simulink model "Flight_Simulation"  (R2021b)
settings: Solver=ode4  StartTime=0.0  StopTime=20  FixedStep=Settings.Simulation.step_size  RelTol=1e-3  EnableMultiTasking=on
undefined symbols (not defined in the file or in its folder): AeroCoeff, Aircraft, ControlGains, dLEF, Environment, F, Light, MIL, Settings, Trim, trim_control, trim_state, trim_thrust
libraries: simulink x19, simulink_extras x14, slpidlib x2, aerolibfltsims x2, aerolibwind2 x1, vrlib x1
(part 2 of 5)

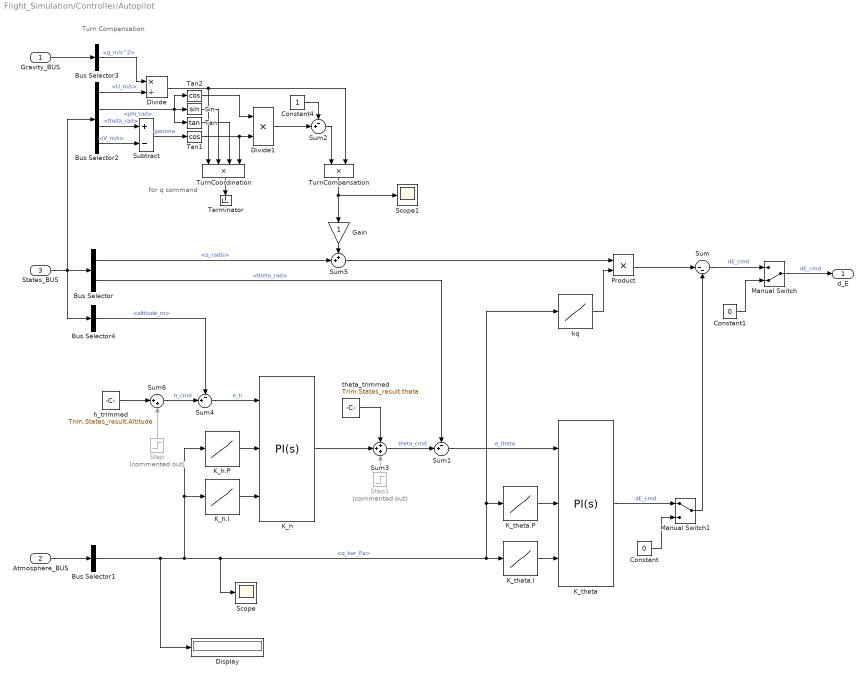
== system Flight_Simulation/Controller/Autopilot ==
  note: for q command
  note: Turn Compensation
  Gravity_BUS : Inport
  Atmosphere_BUS : Inport  Port=2
  States_BUS : Inport  Port=3
  Bus Selector : BusSelector  OutputSignals=Rates_p_q_r.q_rad/s,Angles_phi_theta_psi.theta_rad
  Bus Selector1 : BusSelector  OutputSignals=q_bar_Pa
  Bus Selector2 : BusSelector  OutputSignals=Vel_U_V_W_body.U_m/s,Angles_phi_theta_psi.phi_rad,Angles_phi_theta_psi.theta_rad,Vel_U_V_W_body.V_m/s
  Bus Selector3 : BusSelector  OutputSignals=g_m/s^2
  Bus Selector4 : BusSelector  OutputSignals=Position_north_east_alt.altitude_m
  Constant : Constant  Value=0
  Constant1 : Constant  Value=0
  Constant4 : Constant
  Display : Display
  Divide : Product  Inputs=*/
  Divide1 : Product  Inputs=**
  Gain : Gain
  K_h : slpidlib/PID Controller  Controller=PI  Form=Parallel  TimeDomain=Continuous-time  UseExternalTs=off  SampleTime=-1  IntegratorMethod=Forward Euler  FilterMethod=Forward Euler  ControllerParametersSource=external  P=1  I=1  D=0  UseFilter=on  N=100  TunerSelectOption=Transfer Function Based (PID Tuner App)  InitialConditionSource=internal  InitialConditionForIntegrator=0  InitialConditionForFilter=0  DifferentiatorICPrevScaledInput=0  ExternalReset=none  TrackingMode=off  Kt=1  LimitOutput=off  SatLimitsSource=internal  UpperSaturationLimit=inf  LowerSaturationLimit=-inf  LinearizeAsGain=on  AntiWindupMode=none  Kb=1  POutMin=[]  POutMax=[]  IOutMin=[]  IOutMax=[]  DOutMin=[]  DOutMax=[]  NOutMin=[]  NOutMax=[]  SumOutMin=[]  SumOutMax=[]  SaturationOutMin=[]  SaturationOutMax=[]  PParamMin=[]  PParamMax=[]  IParamMin=[]  IParamMax=[]  DParamMin=[]  DParamMax=[]  NParamMin=[]  NParamMax=[]  KbParamMin=[]  KbParamMax=[]  KtParamMin=[]  KtParamMax=[]  KbOutMin=[]  KbOutMax=[]  KtOutMin=[]  KtOutMax=[]  IntegratorOutMin=[]  IntegratorOutMax=[]  FilterOutMin=[]  FilterOutMax=[]  SumI1OutMin=[]  SumI1OutMax=[]  SumI2OutMin=[]  SumI2OutMax=[]  SumI3OutMin=[]  SumI3OutMax=[]  SumI4OutMin=[]  SumI4OutMax=[]  SumDOutMin=[]  SumDOutMax=[]  DifferentiatorOutMin=[]  DifferentiatorOutMax=[]  FilterDiffOutCoefMin=[]  FilterDiffOutCoefMax=[]  ReciprocalOutMin=[]  ReciprocalOutMax=[]  SumDenOutMin=[]  SumDenOutMax=[]  SumNumOutMin=[]  SumNumOutMax=[]  DivideOutMin=[]  DivideOutMax=[]  UdiffTsProdOutMin=[]  UdiffTsProdOutMax=[]  NTsProdOutMin=[]  NTsProdOutMax=[]  UintegralTsProdOutMin=[]  UintegralTsProdOutMax=[]  UngainTsProdOutMin=[]  UngainTsProdOutMax=[]  IntegratorContinuousStateAttributes=''  IntegratorStateMustResolveToSignalObject=off  IntegratorRTWStateStorageClass=Auto  FilterContinuousStateAttributes=''  FilterStateMustResolveToSignalObject=off  FilterRTWStateStorageClass=Auto  ParallelPVariant=ExternalParameters  IdealPVariant=Disabled  IVariant=ExternalParameters  DVariant=Disabled  IntegratorVariant=Continuous  SatVariant=Disabled  AWVariant=Passthrough  PCopyVariant=Disabled  TRVariant=Disabled  FdbkBlocksVariant=Forward  IdealPFdbkVariant=Disabled  SatFdbkVariant=Disabled  DerivativeFilterVariant=Disabled  NVariant=Disabled  NCopyVariant=Disabled_SignalSpec  FilterICVariant=Disabled  IntegratorICVariant=InternalICs  ExternalResetVariant=Disabled  TRSumVariant=Passthrough  SumFdbkVariant=Disabled  SumVariant=Sum_PI  TsampFilterVariant=InternalTs  TsampNgainVariant=Passthrough  TsampIntegralVariant=Passthrough  ExternalSaturationOutDataTypeStr=Inherit: Same as second input
  K_h.I : Lookup_n-D  NumberOfTableDimensions=1  BreakpointsForDimension1=ControlGains.Schedule  Table=ControlGains.K_h.I  InternalRulePriority=Speed  RndMeth=Simplest  InputSameDT=on
  K_h.P : Lookup_n-D  NumberOfTableDimensions=1  BreakpointsForDimension1=ControlGains.Schedule  Table=ControlGains.K_h.P  InternalRulePriority=Speed  RndMeth=Simplest  InputSameDT=on
  K_theta : slpidlib/PID Controller  Controller=PI  Form=Parallel  TimeDomain=Continuous-time  UseExternalTs=off  SampleTime=-1  IntegratorMethod=Forward Euler  FilterMethod=Forward Euler  ControllerParametersSource=external  P=1  I=1  D=0  UseFilter=on  N=100  TunerSelectOption=Transfer Function Based (PID Tuner App)  InitialConditionSource=internal  InitialConditionForIntegrator=0  InitialConditionForFilter=0  DifferentiatorICPrevScaledInput=0  ExternalReset=none  TrackingMode=off  Kt=1  LimitOutput=off  SatLimitsSource=internal  UpperSaturationLimit=inf  LowerSaturationLimit=-inf  LinearizeAsGain=on  AntiWindupMode=none  Kb=1  POutMin=[]  POutMax=[]  IOutMin=[]  IOutMax=[]  DOutMin=[]  DOutMax=[]  NOutMin=[]  NOutMax=[]  SumOutMin=[]  SumOutMax=[]  SaturationOutMin=[]  SaturationOutMax=[]  PParamMin=[]  PParamMax=[]  IParamMin=[]  IParamMax=[]  DParamMin=[]  DParamMax=[]  NParamMin=[]  NParamMax=[]  KbParamMin=[]  KbParamMax=[]  KtParamMin=[]  KtParamMax=[]  KbOutMin=[]  KbOutMax=[]  KtOutMin=[]  KtOutMax=[]  IntegratorOutMin=[]  IntegratorOutMax=[]  FilterOutMin=[]  FilterOutMax=[]  SumI1OutMin=[]  SumI1OutMax=[]  SumI2OutMin=[]  SumI2OutMax=[]  SumI3OutMin=[]  SumI3OutMax=[]  SumI4OutMin=[]  SumI4OutMax=[]  SumDOutMin=[]  SumDOutMax=[]  DifferentiatorOutMin=[]  DifferentiatorOutMax=[]  FilterDiffOutCoefMin=[]  FilterDiffOutCoefMax=[]  ReciprocalOutMin=[]  ReciprocalOutMax=[]  SumDenOutMin=[]  SumDenOutMax=[]  SumNumOutMin=[]  SumNumOutMax=[]  DivideOutMin=[]  DivideOutMax=[]  UdiffTsProdOutMin=[]  UdiffTsProdOutMax=[]  NTsProdOutMin=[]  NTsProdOutMax=[]  UintegralTsProdOutMin=[]  UintegralTsProdOutMax=[]  UngainTsProdOutMin=[]  UngainTsProdOutMax=[]  IntegratorContinuousStateAttributes=''  IntegratorStateMustResolveToSignalObject=off  IntegratorRTWStateStorageClass=Auto  FilterContinuousStateAttributes=''  FilterStateMustResolveToSignalObject=off  FilterRTWStateStorageClass=Auto  ParallelPVariant=ExternalParameters  IdealPVariant=Disabled  IVariant=ExternalParameters  DVariant=Disabled  IntegratorVariant=Continuous  SatVariant=Disabled  AWVariant=Passthrough  PCopyVariant=Disabled  TRVariant=Disabled  FdbkBlocksVariant=Forward  IdealPFdbkVariant=Disabled  SatFdbkVariant=Disabled  DerivativeFilterVariant=Disabled  NVariant=Disabled  NCopyVariant=Disabled_SignalSpec  FilterICVariant=Disabled  IntegratorICVariant=InternalICs  ExternalResetVariant=Disabled  TRSumVariant=Passthrough  SumFdbkVariant=Disabled  SumVariant=Sum_PI  TsampFilterVariant=InternalTs  TsampNgainVariant=Passthrough  TsampIntegralVariant=Passthrough  ExternalSaturationOutDataTypeStr=Inherit: Same as second input
  K_theta.I : Lookup_n-D  NumberOfTableDimensions=1  BreakpointsForDimension1=ControlGains.Schedule  Table=ControlGains.K_theta.I  InternalRulePriority=Speed  RndMeth=Simplest  InputSameDT=on
  K_theta.P : Lookup_n-D  NumberOfTableDimensions=1  BreakpointsForDimension1=ControlGains.Schedule  Table=ControlGains.K_theta.P  InternalRulePriority=Speed  RndMeth=Simplest  InputSameDT=on
  Manual Switch : ManualSwitch  CurrentSetting=0
  Manual Switch1 : ManualSwitch
  Product : Product
  Scope : Scope
  Scope1 : Scope
  Sin : Trigonometry
  Step : Step  Commented=on  Time=5  After=10  SampleTime=0
  Step1 : Step  Commented=on  Time=5  After=1*pi/180  SampleTime=0
  Subtract : Sum  Inputs=+-
  Sum : Sum  Inputs=|--
  Sum1 : Sum  Inputs=-+|
  Sum2 : Sum  Inputs=-+|
  Sum3 : Sum  Inputs=+++
  Sum4 : Sum  Inputs=-+|
  Sum5 : Sum  Inputs=++|
  Sum6 : Sum  Inputs=|++
  Tan : Trigonometry  Operator=tan
  Tan1 : Trigonometry  Operator=cos
  Tan2 : Trigonometry  Operator=cos
  Terminator : Terminator
  TurnCompensation : Product
  TurnCoordination : Product  Inputs=4
  h_trimmed : Constant  Value=Trim.States_result.Altitude
  kq : Lookup_n-D  NumberOfTableDimensions=1  BreakpointsForDimension1=ControlGains.Schedule  Table=ControlGains.kq  InternalRulePriority=Speed  RndMeth=Simplest  InputSameDT=on
  theta_trimmed : Constant  Value=Trim.States_result.theta
  d_E : Outport
  wires:
  States_BUS/1 -> Bus Selector2/1, Bus Selector4/1, Bus Selector/1
  Product/1 -> Sum/1
  Manual Switch/1 -> d_E/1  "dE_cmd"
  Sum/1 -> Manual Switch/1  "dE_cmd"
  Constant/1 -> Manual Switch1/2
  Manual Switch1/1 -> Sum/2
  Constant1/1 -> Manual Switch/2
  Sum1/1 -> K_theta/1  "e_theta"
  Bus Selector2/1 -> Divide/2  "<U_m/s>"
  Gravity_BUS/1 -> Bus Selector3/1
  Bus Selector3/1 -> Divide/1  "<g_m/s^2>"
  Divide/1 -> TurnCompensation/2, TurnCoordination/1
  Bus Selector2/2 -> Tan2/1, Sin/1, Tan/1  "<phi_rad>"
  Bus Selector2/4 -> Subtract/2  "<V_m/s>"
  Bus Selector2/3 -> Subtract/1  "<theta_rad>"
  TurnCoordination/1 -> Terminator/1
  Step1/1 -> Sum3/3
  Subtract/1 -> Tan1/1  "gamma"
  Tan1/1 -> Divide1/2, TurnCoordination/4
  Tan/1 -> TurnCoordination/3
  Sin/1 -> TurnCoordination/2
  Atmosphere_BUS/1 -> Bus Selector1/1
  theta_trimmed/1 -> Sum3/1
  Bus Selector4/1 -> Sum4/1  "<altitude_m>"
  h_trimmed/1 -> Sum6/1
  Sum4/1 -> K_h/1  "e_h"
  Step/1 -> Sum6/2
  Bus Selector/1 -> Sum5/2  "<q_rad/s>"
  Bus Selector/2 -> Sum1/1  "<theta_rad>"
  Constant4/1 -> Sum2/1
  Divide1/1 -> Sum2/2
  Sum2/1 -> TurnCompensation/1
  Sum5/1 -> Product/1
  Tan2/1 -> Divide1/1
  TurnCompensation/1 -> Gain/1, Scope1/1
  K_theta/1 -> Manual Switch1/1  "dE_cmd"
  K_h/1 -> Sum3/2
  Sum3/1 -> Sum1/2  "theta_cmd"
  Sum6/1 -> Sum4/2  "h_cmd"
  Bus Selector1/1 -> Display/1, K_h.I/1, K_h.P/1, Scope/1, kq/1, K_theta.P/1, K_theta.I/1  "<q_bar_Pa>"
  kq/1 -> Product/2
  K_h.P/1 -> K_h/2
  K_h.I/1 -> K_h/3
  K_theta.P/1 -> K_theta/2
  K_theta.I/1 -> K_theta/3
  Gain/1 -> Sum5/1

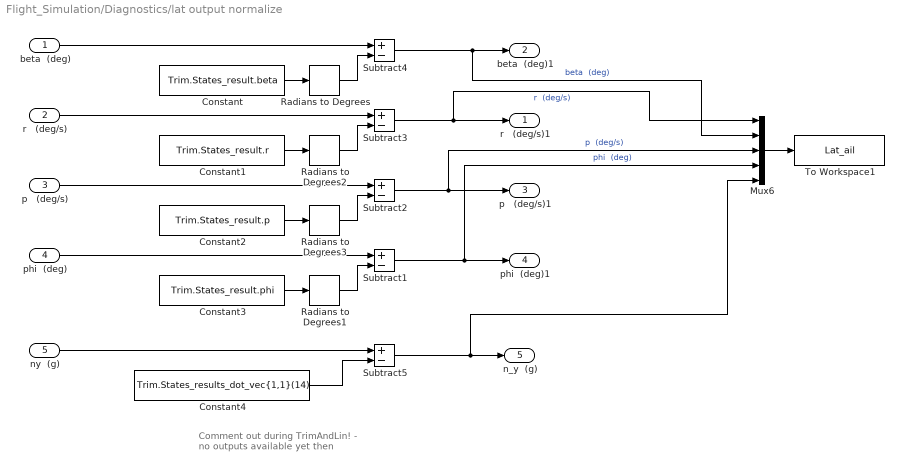
== system Flight_Simulation/Diagnostics/lat output normalize ==
  note: Comment out during TrimAndLin!
      | - no outputs available yet then
  beta  (deg) : Inport
  r   (deg/s) : Inport  Port=2
  p   (deg/s) : Inport  Port=3
  phi  (deg) : Inport  Port=4
  ny  (g) : Inport  Port=5
  Constant : Constant  Value=Trim.States_result.beta
  Constant1 : Constant  Value=Trim.States_result.r
  Constant2 : Constant  Value=Trim.States_result.p
  Constant3 : Constant  Value=Trim.States_result.phi
  Constant4 : Constant  Value=Trim.States_results_dot_vec{1,1}(14)
  Mux6 : Mux  Inputs=5
  Radians to Degrees{,1..3} (4 alike) : simulink_extras/Transformations/Radians to Degrees
  Subtract{1..5} (5 alike) : Sum  Inputs=+-
  To Workspace1 : ToWorkspace  VariableName=Lat_ail  SampleTime=-1
  r   (deg/s)1 : Outport
  beta  (deg)1 : Outport  Port=2
  p   (deg/s)1 : Outport  Port=3
  phi  (deg)1 : Outport  Port=4
  n_y  (g) : Outport  Port=5
  wires:
  beta  (deg)/1 -> Subtract4/1
  p   (deg/s)/1 -> Subtract2/1
  r   (deg/s)/1 -> Subtract3/1
  phi  (deg)/1 -> Subtract1/1
  Constant/1 -> Radians to Degrees/1
  Constant1/1 -> Radians to Degrees2/1
  Constant2/1 -> Radians to Degrees3/1
  Constant3/1 -> Radians to Degrees1/1
  Radians to Degrees/1 -> Subtract4/2
  Radians to Degrees2/1 -> Subtract3/2
  Radians to Degrees3/1 -> Subtract2/2
  Radians to Degrees1/1 -> Subtract1/2
  Constant4/1 -> Subtract5/2
  ny  (g)/1 -> Subtract5/1
  Subtract4/1 -> Mux6/2, beta  (deg)1/1  "beta  (deg)"
  Subtract3/1 -> Mux6/1, r   (deg/s)1/1  "r  (deg/s)"
  Subtract1/1 -> Mux6/4, phi  (deg)1/1  "phi  (deg)"
  Subtract2/1 -> Mux6/3, p   (deg/s)1/1  "p  (deg/s)"
  Mux6/1 -> To Workspace1/1
  Subtract5/1 -> Mux6/5, n_y  (g)/1

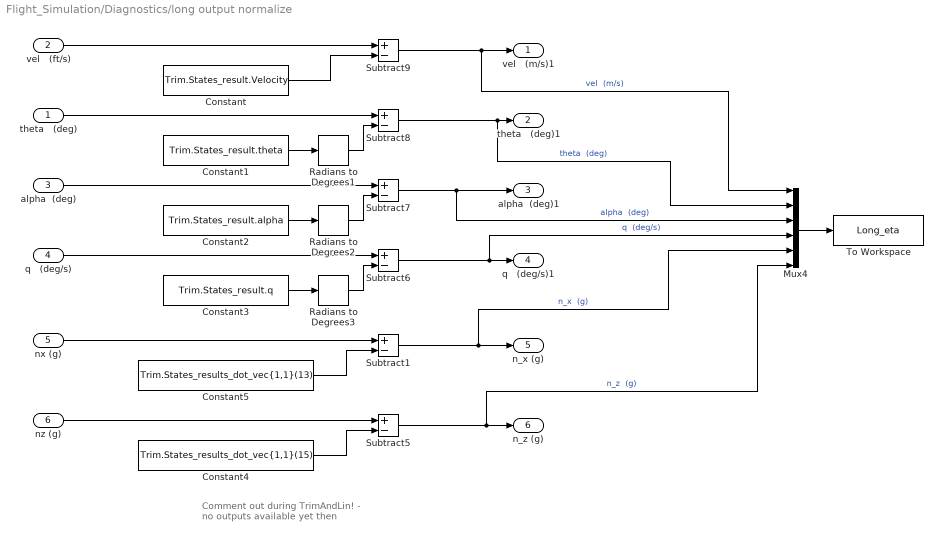
== system Flight_Simulation/Diagnostics/long output normalize ==
  note: Comment out during TrimAndLin!
      | - no outputs available yet then
  theta   (deg) : Inport
  vel   (ft/s) : Inport  Port=2
  alpha  (deg) : Inport  Port=3
  q   (deg/s) : Inport  Port=4
  nx (g) : Inport  Port=5
  nz (g) : Inport  Port=6
  Constant : Constant  Value=Trim.States_result.Velocity
  Constant1 : Constant  Value=Trim.States_result.theta
  Constant2 : Constant  Value=Trim.States_result.alpha
  Constant3 : Constant  Value=Trim.States_result.q
  Constant4 : Constant  Value=Trim.States_results_dot_vec{1,1}(15)
  Constant5 : Constant  Value=Trim.States_results_dot_vec{1,1}(13)
  Mux4 : Mux  Inputs=6
  Radians to Degrees1 : simulink_extras/Transformations/Radians to Degrees
  Radians to Degrees2 : simulink_extras/Transformations/Radians to Degrees
  Radians to Degrees3 : simulink_extras/Transformations/Radians to Degrees
  Subtract{1,5..9} (6 alike) : Sum  Inputs=+-
  To Workspace : ToWorkspace  VariableName=Long_eta  SampleTime=-1
  vel   (m/s)1 : Outport
  theta   (deg)1 : Outport  Port=2
  alpha  (deg)1 : Outport  Port=3
  q   (deg/s)1 : Outport  Port=4
  n_x (g) : Outport  Port=5
  n_z (g) : Outport  Port=6
  wires:
  vel   (ft/s)/1 -> Subtract9/1
  alpha  (deg)/1 -> Subtract7/1
  theta   (deg)/1 -> Subtract8/1
  nz (g)/1 -> Subtract5/1
  q   (deg/s)/1 -> Subtract6/1
  Constant/1 -> Subtract9/2
  Constant1/1 -> Radians to Degrees1/1
  Constant2/1 -> Radians to Degrees2/1
  Constant3/1 -> Radians to Degrees3/1
  Constant4/1 -> Subtract5/2
  Radians to Degrees1/1 -> Subtract8/2
  Radians to Degrees2/1 -> Subtract7/2
  Radians to Degrees3/1 -> Subtract6/2
  Constant5/1 -> Subtract1/2
  nx (g)/1 -> Subtract1/1
  Subtract7/1 -> Mux4/3, alpha  (deg)1/1  "alpha  (deg)"
  Subtract5/1 -> Mux4/6, n_z (g)/1  "n_z  (g)"
  Subtract8/1 -> Mux4/2, theta   (deg)1/1  "theta  (deg)"
  Mux4/1 -> To Workspace/1
  Subtract1/1 -> Mux4/5, n_x (g)/1  "n_x  (g)"
  Subtract6/1 -> Mux4/4, q   (deg/s)1/1  "q  (deg/s)"
  Subtract9/1 -> Mux4/1, vel   (m/s)1/1  "vel  (m/s)"

== system Flight_Simulation/Environment_Subsystems/Earth_Model ==
  States_BUS : Inport
  Bus Creator : BusCreator  Inputs=3
  Bus Selector : BusSelector  OutputSignals=Pos_WGS84.mue_pos_WGS84_rad
  Constant : Constant
  Earth_Radius_m : Constant  Value=6371000
  Earth_rotation_rate_rad/s : Constant  Commented=on  Value=7.2921150e-5
  Math Function : Math  Operator=square  SignedPower=on  SaturateOnIntegerOverflow=on
  Product : Product
  Product1 : Product  Inputs=*/
  Product2 : Product  Inputs=*/*
  Semi_major_axis_m : Constant  Value=6378137
  Sqrt : Sqrt  SaturateOnIntegerOverflow=on
  Sum : Sum  Inputs=|-+
  Sum1 : Sum  Inputs=+-|
  Terminator : Terminator
  Trigonometric Function : Trigonometry
  first_excentricity_squared : Constant  Value=6.69437999014*10^(-3)
  Earth_Model_BUS : Outport
  wires:
  Trigonometric Function/1 -> Math Function/1
  Math Function/1 -> Product/1
  first_excentricity_squared/1 -> Sum1/2, Product/2
  Product/1 -> Sum/1
  Constant/1 -> Sum1/1, Sum/2
  Sum/1 -> Product2/2, Sqrt/1
  Sqrt/1 -> Product1/2
  Semi_major_axis_m/1 -> Product1/1
  Sum1/1 -> Product2/3
  Product1/1 -> Product2/1, Bus Creator/1  "R_Curvature_Prime_Vertical_m"
  Earth_Radius_m/1 -> Terminator/1  "round_earth"
  Product2/1 -> Bus Creator/2  "R_Curvature_Meridian_m"
  Bus Creator/1 -> Earth_Model_BUS/1  "Earth_Model_BUS"
  Earth_rotation_rate_rad/s/1 -> Bus Creator/3  "Earth_rotation_rate_rad/s"
  States_BUS/1 -> Bus Selector/1  "Pos_mue_WGS84"
  Bus Selector/1 -> Trigonometric Function/1  "<mue_pos_WGS84_rad>"

== system Flight_Simulation/Environment_Subsystems/Gravity_Model_simple ==
  States_BUS : Inport
  Bus Creator : BusCreator  Inputs=1
  Terminator : Terminator
  g : Constant  Value=Environment.Const.g0
  Gravity_BUS : Outport
  wires:
  States_BUS/1 -> Terminator/1
  g/1 -> Bus Creator/1  "g_m/s^2"
  Bus Creator/1 -> Gravity_BUS/1  "Gravity_BUS"

== system Flight_Simulation/Environment_Subsystems/ISA_StandardAtmosphere_Model_ScriptVersion ==
  States_BUS : Inport
  Gravity_BUS : Inport  Port=2
  Vel_Aero_BUS : Inport  Port=3
  Bus Creator : BusCreator  Inputs=5
  Bus Selector : BusSelector  OutputSignals=Position_north_east_alt.altitude_m
  Bus Selector1 : BusSelector  OutputSignals=g_m/s^2
  Bus Selector2 : BusSelector  OutputSignals=Vel_aero_V_alpha_beta.v_m/s
  Compressibility_Setting : Constant  Value=Settings.Compressibility
  ISA_Standard_Atmosphere_Model : MATLAB Function  TreatAsAtomicUnit=on
  R : Constant  Value=Environment.Const.R
  Atmosphere_BUS : Outport
  wires:
  States_BUS/1 -> Bus Selector/1
  Bus Creator/1 -> Atmosphere_BUS/1  "Atmosphere_BUS"
  Bus Selector/1 -> ISA_Standard_Atmosphere_Model/1(H)  "<altitude_m>"
  Gravity_BUS/1 -> Bus Selector1/1
  Bus Selector1/1 -> ISA_Standard_Atmosphere_Model/3(g)  "<g_m/s^2>"
  ISA_Standard_Atmosphere_Model/3(rho) -> Bus Creator/3  "rho_kg/m^3"
  ISA_Standard_Atmosphere_Model/4(T) -> Bus Creator/4  "T_K"
  ISA_Standard_Atmosphere_Model/5(Mach) -> Bus Creator/5  "Mach"
  ISA_Standard_Atmosphere_Model/2(q_bar) -> Bus Creator/2  "q_bar_Pa"
  ISA_Standard_Atmosphere_Model/1(p_static) -> Bus Creator/1  "p_static_Pa"
  R/1 -> ISA_Standard_Atmosphere_Model/4(R)
  Compressibility_Setting/1 -> ISA_Standard_Atmosphere_Model/5(compressibility)
  Vel_Aero_BUS/1 -> Bus Selector2/1
  Bus Selector2/1 -> ISA_Standard_Atmosphere_Model/2(V)  "<v_m/s>"

== system Flight_Simulation/Environment_Subsystems/ISA_StandardAtmosphere_Model_SimulinkVersion ==
  note: to be updated
  States_BUS : Inport
  Gravity_BUS : Inport  Port=2
  Vel_aero_BUS : Inport  Port=3
  Bus Creator : BusCreator  Inputs=5
  Bus Selector : BusSelector  OutputSignals=Position_north_east_alt.altitude_m
  Bus Selector1 : BusSelector  OutputSignals=g_m/s^2
  Bus Selector2 : BusSelector  OutputSignals=Vel_aero_V_alpha_beta.v_m/s
  Constants depending on Height : Subsystem
  Divide1 : Product  Inputs=/*
  Gain : Gain  Gain=-1
  Height flags : Subsystem
  Mach : Subsystem
  T : Subsystem
  p_static : Subsystem
  q_bar : Subsystem
  rho : Subsystem
  Atmosphere_BUS : Outport
  wires:
  States_BUS/1 -> Bus Selector/1
  Bus Selector/1 -> Height flags/1(altitude), Constants depending on Height/1(altitude)  "<altitude_m>"
  Bus Creator/1 -> Atmosphere_BUS/1  "Atmosphere_BUS"
  Bus Selector2/1 -> q_bar/3(v), Mach/3(v)  "<v_m/s>"
  p_static/1(p) -> q_bar/1(p_static), Bus Creator/1  "p_static_Pa"
  Height flags/1(Height_flg) -> T/3(Height_flg), p_static/6(Height_flg), rho/6(Height_flg), Constants depending on Height/2(Height_flg)
  Constants depending on Height/5((H - H_A)*beta) -> T/1((H - H_A)*beta), rho/4((H - H_A)*beta), p_static/4((H - H_A)*beta)
  Mach/1(Mach) -> q_bar/4(Mach), Bus Creator/5  "Mach"
  q_bar/1(q_bar) -> Bus Creator/2  "q_bar_Pa"
  T/1(T) -> Bus Creator/4, Mach/1(T)  "T_K"
  rho/1(rho) -> Bus Creator/3, q_bar/2(rho)  "rho_kg/m^3"
  Constants depending on Height/4(H - H_A) -> p_static/3(H - H_A), rho/3(H - H_A)
  Gravity_BUS/1 -> Bus Selector1/1
  Bus Selector1/1 -> Divide1/2  "<g_m/s^2>"
  Divide1/1 -> Gain/1  "g/R"
  Gain/1 -> p_static/7(-g/R), rho/7(-g/R)  "-g/R"
  Constants depending on Height/6(T_A) -> p_static/5(T_A), T/2(T_A), rho/5(T_A)
  Constants depending on Height/1(p_A) -> p_static/1(p_A)
  Constants depending on Height/7(R) -> Mach/2(R), Divide1/1
  Constants depending on Height/2(rho_A) -> rho/1(rho_A)
  Constants depending on Height/3(beta) -> p_static/2(beta), rho/2(beta)
  Vel_aero_BUS/1 -> Bus Selector2/1

== system Flight_Simulation/Environment_Subsystems/Wind_Input ==
  States_BUS : Inport
  Wind_BUS : Inport  Port=2
  Flag_Settings_BUS : Inport  Port=3
  Const_Wind_Vel_UVWe_m/s : Inport  Port=4
  Bus Creator : BusCreator  Inputs=2
  Bus Creator1 : BusCreator  Inputs=3
  Bus Selector : BusSelector  OutputSignals=Angles_phi_theta_psi,Vel_U_V_W_body
  Bus Selector1 : BusSelector  OutputSignals=u_wind_m/s,v_wind_m/s,w_wind_m/s
  Bus Selector2 : BusSelector  OutputSignals=U_m/s,V_m/s,W_m/s
  Bus Selector3 : BusSelector  OutputSignals=phi_rad,theta_rad,psi_rad
  Bus Selector4 : BusSelector  OutputSignals=const_u_wind_m/s,const_v_wind_m/s,const_w_wind_m/s
  Bypass for TrimAndLin : Subsystem
  Calc_Vel_aero_alpha_beta : Subsystem
  Sum : Sum  Inputs=-+|
  Sum1 : Sum  Inputs=-+|
  Sum2 : Sum  Inputs=++|
  Sum3 : Sum  Inputs=++|
  Sum4 : Sum  Inputs=++|
  Sum5 : Sum  Inputs=-+|
  wind earth2body trafo : MATLAB Function  TreatAsAtomicUnit=on
  Vel_aero_BUS : Outport
  wires:
  States_BUS/1 -> Bus Selector/1
  Bus Selector/1 -> Bus Selector3/1  "<Angles_phi_theta_psi>"
  Bus Creator/1 -> Vel_aero_BUS/1  "Vel_aero_BUS"
  Wind_BUS/1 -> Bypass for TrimAndLin/1(Wind_BUS)
  Bus Selector1/1 -> Sum3/2  "<u_wind_m/s>"
  Bus Selector1/2 -> Sum4/2  "<v_wind_m/s>"
  Bus Selector1/3 -> Sum2/2  "<w_wind_m/s>"
  Bus Selector3/1 -> wind earth2body trafo/4(phi)  "<phi_rad>"
  Bus Selector3/2 -> wind earth2body trafo/5(theta)  "<theta_rad>"
  Bus Selector3/3 -> wind earth2body trafo/6(psi)  "<psi_rad>"
  Const_Wind_Vel_UVWe_m/s/1 -> Bus Selector4/1
  Bus Selector4/3 -> Sum2/1  "<const_w_wind_m/s>"
  Bus Selector4/2 -> Sum4/1  "<const_v_wind_m/s>"
  Bus Selector4/1 -> Sum3/1  "<const_u_wind_m/s>"
  Sum3/1 -> wind earth2body trafo/1(Ue)
  Sum4/1 -> wind earth2body trafo/2(Ve)
  Sum2/1 -> wind earth2body trafo/3(We)
  Bus Selector2/1 -> Sum/2  "<U_m/s>"
  Bus Selector2/2 -> Sum1/2  "<V_m/s>"
  Sum/1 -> Bus Creator1/1  "U_aero_m/s"
  Sum1/1 -> Bus Creator1/2  "V_aero_m/s"
  Sum5/1 -> Bus Creator1/3  "W_aero_m/s"
  Bus Creator1/1 -> Calc_Vel_aero_alpha_beta/1(Vel_U_V_W_BUS), Bus Creator/2  "Vel_U_V_W_aero"
  Calc_Vel_aero_alpha_beta/1(Vel_aero_alpha_beta_BUS) -> Bus Creator/1  "Vel_aero_V_alpha_beta"
  Bus Selector/2 -> Bus Selector2/1  "<Vel_U_V_W_body>"
  Bus Selector2/3 -> Sum5/2  "<W_m/s>"
  Bypass for TrimAndLin/1(Wind_Vel) -> Bus Selector1/1  "Wind_Vel_UVWe_m/s"
  Flag_Settings_BUS/1 -> Bypass for TrimAndLin/2(Flag_Settings_BUS)
  wind earth2body trafo/3(Ww) -> Sum5/1
  wind earth2body trafo/2(Vw) -> Sum1/1
  wind earth2body trafo/1(Uw) -> Sum/1

== system Flight_Simulation/Environment_Subsystems/Wind_Model ==
  note: because transformation is already done
      | in the wind input block
  note: A selfmade turbulence model has yet to be implemented!
  Atmosphere_BUS : Inport
  States_BUS : Inport  Port=2
  Aircraft_Constants_BUS : Inport  Port=3
  Bus Selector : BusSelector  OutputSignals=Position_north_east_alt.altitude_m,Vel_U_V_W_body.U_m/s
  Bus Selector1 : BusSelector  OutputSignals=FlightProfileAlleviationFactor_Fg
  Constant : Constant  Value=ones(3,3)
  Demux : Demux  Outputs=3
  Demux1 : Demux  Outputs=3
  Dryden Wind Turbulence Model (Discrete (+q +r)) : aerolibwind2/Dryden Wind Turbulence Model  (Continuous (+q -r))  Commented=on  units=Metric (MKS)  spec=MIL-F-8785C  model=Discrete Dryden (+q +r)  W20=15  Wdeg=0  TurbProb=10^-2 - Light  L_high=533.4  Wingspan=Aircraft.Dimensions.MAC  ts=0.1  Seed=[23341 23342 23343 23344]  T_on=off
  Gust_model_(1-cos) : Subsystem
      mask Display: image('1-cos-gust.png'); % Use "Edit Image" on toolstrip to change.
  Mux1 : Mux  Inputs=3
  Sum : Sum  Inputs=+++
  Sum1 : Sum  Inputs=+++
  Sum2 : Sum  Inputs=+++
  Terminator : Terminator
  simple step gust : Step  Time=Environment.gust.steptimes  After=Environment.gust.step_amplitude  SampleTime=0
  Wind_BUS : Outport
  wires:
  States_BUS/1 -> Bus Selector/1
  Mux1/1 -> Wind_BUS/1  "Wind_Vel_UVWe_m/s"
  Aircraft_Constants_BUS/1 -> Bus Selector1/1
  Bus Selector1/1 -> Gust_model_(1-cos)/2(FlightProfileAlleviationFactor_Fg)  "<FlightProfileAlleviationFactor_Fg>"
  Bus Selector/1 -> Dryden Wind Turbulence Model (Discrete (+q +r))/1, Gust_model_(1-cos)/3(altitude_m)  "<altitude_m>"
  Bus Selector/2 -> Dryden Wind Turbulence Model (Discrete (+q +r))/2, Gust_model_(1-cos)/4(v_m/s)  "<U_m/s>"
  Sum/1 -> Mux1/1  "u_wind_m/s"
  Sum1/1 -> Mux1/2  "v_wind_m/s"
  Sum2/1 -> Mux1/3  "w_wind_m/s"
  Gust_model_(1-cos)/1(u_wind_m/s) -> Sum/2
  simple step gust/1 -> Demux/1
  Demux/1 -> Sum/1
  Demux/2 -> Sum1/1
  Demux/3 -> Sum2/1
  Dryden Wind Turbulence Model (Discrete (+q +r))/1 -> Demux1/1
  Demux1/1 -> Sum/3
  Demux1/2 -> Sum1/3
  Demux1/3 -> Sum2/3
  Gust_model_(1-cos)/3(w_wind_m/s) -> Sum2/2
  Gust_model_(1-cos)/2(v_wind_m/s) -> Sum1/2
  Constant/1 -> Dryden Wind Turbulence Model (Discrete (+q +r))/3
  Dryden Wind Turbulence Model (Discrete (+q +r))/2 -> Terminator/1
  Atmosphere_BUS/1 -> Gust_model_(1-cos)/1(Atmosphere_BUS)

== system Flight_Simulation/Input_BusCreation/Evaluate Joystick Input ==
  Aircraft_Constants_BUS : Inport
  Flag_Settings_BUS : Inport  Port=2
  Joystick : Inport  Port=3
  1-D Lookup Table : Lookup_n-D  NumberOfTableDimensions=1  BreakpointsForDimension1=[-1,1]  TableSource=Input port  Table=tanh([-5:5])  InternalRulePriority=Speed  RndMeth=Simplest  InputSameDT=on
      settings: InputPortMap=u0,p221
  Abs1 : Abs
  Abs2 : Abs
  Bus Selector : BusSelector  OutputSignals=Control_Surface_Const_BUS.Aileron_BUS.Ail_pos_min_deg,Control_Surface_Const_BUS.Aileron_BUS.Ail_pos_max_deg
  Bus Selector1 : BusSelector  OutputSignals=Control_Surface_Const_BUS.Elevator_BUS.Elev_pos_min_deg,Control_Surface_Const_BUS.Elevator_BUS.Elev_pos_max_deg
  Bus Selector2 : BusSelector  OutputSignals=Engine_Const_BUS.thrust_max,Engine_Const_BUS.thrust_min
  Bus Selector3 : BusSelector  OutputSignals=Linearization_Flag,Trim_Flag
  Constant : Constant  Value=0
  Demux : Demux  Outputs=3
  Logical Operator : Logic  Operator=OR  AllPortsSameDT=off  OutDataTypeStr=boolean
  Mux : Mux  Inputs=2
  Product{,1..3} (4 alike) : Product
  Selector : Selector  InputPortWidth=8  IndexOptions=Index vector (dialog)  Indices=[1 2 3]  OutputSizes=1
  Switch : Switch
  Switch1 : Switch
  Switch2 : Switch  Criteria=u2 > Threshold
  Joystick_Aileron_deg : Outport
  Joystick_Elevator_deg : Outport  Port=2
  Joystick_Thrust_N : Outport  Port=3
  wires:
  Bus Selector3/2 -> Logical Operator/2  "<Trim_Flag>"
  Bus Selector1/1 -> Product2/1  "<Elev_pos_min_deg>"
  Aircraft_Constants_BUS/1 -> Bus Selector2/1, Bus Selector1/1, Bus Selector/1
  Product1/1 -> Switch/3
  Bus Selector/2 -> Product1/2  "<Ail_pos_max_deg>"
  Bus Selector2/2 -> Mux/2  "<thrust_min>"
  1-D Lookup Table/1 -> Joystick_Thrust_N/1  "Joystick_Thrust_N"
  Bus Selector/1 -> Product/1  "<Ail_pos_min_deg>"
  Abs1/1 -> Product1/1
  Demux/2 -> Abs2/1, Product2/2, Switch1/2  "Elevator_-1..1"
  Flag_Settings_BUS/1 -> Bus Selector3/1
  Mux/1 -> 1-D Lookup Table/2
  Product3/1 -> Switch1/3
  Switch/1 -> Joystick_Aileron_deg/1  "Joystick_Aileron_deg"
  Product/1 -> Switch/1
  Demux/1 -> Product/2, Switch/2, Abs1/1  "Aileron_-1..1"
  Product2/1 -> Switch1/1
  Abs2/1 -> Product3/1
  Switch1/1 -> Joystick_Elevator_deg/1  "Joystick_Elevator_deg"
  Bus Selector2/1 -> Mux/1  "<thrust_max>"
  Bus Selector1/2 -> Product3/2  "<Elev_pos_max_deg>"
  Bus Selector3/1 -> Logical Operator/1  "<Linearization_Flag>"
  Demux/3 -> 1-D Lookup Table/1  "Thrust_-1..1"
  Joystick/1 -> Switch2/3
  Logical Operator/1 -> Switch2/2
  Constant/1 -> Switch2/1
  Switch2/1 -> Selector/1
  Selector/1 -> Demux/1

== system Flight_Simulation/Non-linear_Plant/6DOF_Equations ==
  States_BUS : Inport
  AeroForces_total_BUS : Inport  Port=2
  AeroMoments_total_BUS : Inport  Port=3
  Engine_BUS : Inport  Port=4
  Aircraft_Constants_BUS : Inport  Port=5
  Gravity_BUS : Inport  Port=6
  Earth_Model_BUS : Inport  Port=7
  Acceleration_nx_ny_nz_Calculation : Subsystem
  Attitude_Differential_Equations : Subsystem
  Bus Creator : BusCreator  Inputs=4
  Position_Differential_Equations : Subsystem
  Rotation_Differential_Equation : Subsystem
  Translation_UVW_Differential_Equations : Subsystem
  State_dot_BUS : Outport
  Acc_nx_ny_nz_BUS : Outport  Port=2
  wires:
  Position_Differential_Equations/1(Position_dot_BUS) -> Bus Creator/1
  Attitude_Differential_Equations/1(Attitude_dot_BUS) -> Bus Creator/2
  Aircraft_Constants_BUS/1 -> Rotation_Differential_Equation/1(Aircraft_Constants_BUS), Translation_UVW_Differential_Equations/4(Aircraft_Constants_BUS)
  Gravity_BUS/1 -> Acceleration_nx_ny_nz_Calculation/3(Gravity_BUS), Translation_UVW_Differential_Equations/5(Gravity_BUS)
  Translation_UVW_Differential_Equations/1(Vel_U_V_W_body_dot_BUS) -> Acceleration_nx_ny_nz_Calculation/1(Vel_U_V_W_dot_BUS), Bus Creator/3
  Rotation_Differential_Equation/1(Rates_dot_p_q_r) -> Bus Creator/4
  Bus Creator/1 -> State_dot_BUS/1  "State_dot_BUS"
  Acceleration_nx_ny_nz_Calculation/1(Acc_nx_ny_nz_BUS) -> Acc_nx_ny_nz_BUS/1
  Engine_BUS/1 -> Rotation_Differential_Equation/2(Engine_BUS), Translation_UVW_Differential_Equations/3(Engine_BUS)
  Earth_Model_BUS/1 -> Position_Differential_Equations/1(Earth_Model_BUS)
  AeroForces_total_BUS/1 -> Translation_UVW_Differential_Equations/2(Forces_total_BUS)
  AeroMoments_total_BUS/1 -> Rotation_Differential_Equation/4(Moments_total_BUS)
  States_BUS/1 -> Position_Differential_Equations/2(States_BUS), Attitude_Differential_Equations/1(States_BUS), Acceleration_nx_ny_nz_Calculation/2(States_BUS), Rotation_Differential_Equation/3(States_BUS), Translation_UVW_Differential_Equations/1(States_BUS)

== system Flight_Simulation/Non-linear_Plant/Actuator_Models ==
  note: not implemented yet - from F16 model
  Vel_aero_BUS : Inport
  Command_BUS : Inport  Port=2
  Flag_Settings_BUS : Inport  Port=3
  Init_BUS : Inport  Port=4
  Aircraft_Constants_BUS : Inport  Port=5
  Atmosphere_BUS : Inport  Port=6
  Aileron Actuator : Subsystem
  Bus Creator : BusCreator  Inputs=4
  Bus Selector : BusSelector  OutputSignals=Elevator_cmd_deg,Aileron_cmd_deg,Rudder_cmd_deg,Speedbrakes_cmd_%
  Bus Selector1 : BusSelector  OutputSignals=U_init_BUS.Elevator_init_deg,U_init_BUS.Aileron_init_deg,U_init_BUS.Rudder_init_deg
  Bus Selector2 : BusSelector  OutputSignals=Linearization_Flag
  Bus Selector3 : BusSelector  OutputSignals=Control_Surface_Const_BUS
  Elevator Actuator : Subsystem
  Leading Edge Flap : Subsystem
  Rudder Actuator : Subsystem
  Sum : Sum  Inputs=|++
  Sum1 : Sum  Inputs=|++
  Switch : Switch  Criteria=u2 > Threshold
  Switch1 : Switch  Criteria=u2 > Threshold
  Switch2 : Switch  Criteria=u2 > Threshold
  test : Step  Commented=on  Time=5  After=0.5  SampleTime=0
  test1 : Step  Commented=on  Time=5  After=0.01
  Flaps_BUS : Outport
  Controls_BUS : Outport  Port=2
  wires:
  Elevator Actuator/1(Elevator_act_deg) -> Switch2/3  "Elevator_act_deg"
  Sum/1 -> Bus Creator/2  "Aileron_act_deg"
  Switch/1 -> Bus Creator/3  "Rudder_act_deg"
  Command_BUS/1 -> Bus Selector/1
  Bus Selector/2 -> Switch1/1, Aileron Actuator/1(Aileron_cmd_deg)  "<Aileron_cmd_deg>"
  Bus Selector/1 -> Switch2/1, Elevator Actuator/1(Elevator_cmd_deg)  "<Elevator_cmd_deg>"
  Bus Selector/3 -> Switch/1, Rudder Actuator/1(Rudder_cmd_deg)  "<Rudder_cmd_deg>"
  Bus Creator/1 -> Controls_BUS/1  "Controls_BUS"
  Init_BUS/1 -> Bus Selector1/1
  Bus Selector1/1 -> Elevator Actuator/3(Elevator_init_deg)  "<Elevator_init_deg>"
  Bus Selector1/2 -> Aileron Actuator/3(Aileron_init_deg)  "<Aileron_init_deg>"
  Bus Selector1/3 -> Rudder Actuator/3(Rudder_init_deg)  "<Rudder_init_deg>"
  Sum1/1 -> Bus Creator/1  "Elevator_act_deg"
  Aileron Actuator/1(Aileron_act_deg) -> Switch1/3  "Aileron_act_deg"
  Rudder Actuator/1(Rudder_act_deg) -> Switch/3  "Rudder_act_deg"
  Flag_Settings_BUS/1 -> Bus Selector2/1
  Bus Selector2/1 -> Switch2/2, Switch1/2, Switch/2  "<Linearization_Flag>"
  Leading Edge Flap/1(LE_Flap_deg) -> Flaps_BUS/1  "Flaps_BUS"
  Aircraft_Constants_BUS/1 -> Bus Selector3/1
  Bus Selector3/1 -> Elevator Actuator/2(Control_Surface_Const_BUS), Rudder Actuator/2(Control_Surface_Const_BUS), Aileron Actuator/2(Control_Surface_Const_BUS)  "<Control_Surface_Const_BUS>"
  Atmosphere_BUS/1 -> Leading Edge Flap/1(Atmosphere_BUS)
  Bus Selector/4 -> Bus Creator/4  "<Speedbrakes_cmd_%>"
  Switch1/1 -> Sum/1
  test1/1 -> Sum/2
  Switch2/1 -> Sum1/1
  test/1 -> Sum1/2
  Vel_aero_BUS/1 -> Leading Edge Flap/2(States_BUS)

== system Flight_Simulation/Non-linear_Plant/Aerodynamic_Modul ==
  Atmosphere_BUS : Inport
  States_BUS : Inport  Port=2
  Vel_aero_BUS : Inport  Port=3
  Aircraft_Constant_BUS : Inport  Port=4
  LE_Flaps_BUS : Inport  Port=5
  Controls_BUS : Inport  Port=6
  Engine_BUS : Inport  Port=7
  Aero_Coefficients : Subsystem
  Bus Selector : BusSelector  OutputSignals=X_total,Z_total
  Bus Selector1 : BusSelector  OutputSignals=M_total
  Mux : Mux  Inputs=2
  Scope : Scope
  Scope1 : Scope
  States with Wind : Subsystem
  Terminator : Terminator
  To Workspace : ToWorkspace  Commented=on  VariableName=stepGust_ONERA_Forces  SampleTime=-1
  To Workspace1 : ToWorkspace  Commented=on  VariableName=stepGust_ONERA_Moment  SampleTime=-1
  Total Aero Forces : Subsystem
  Total Aero Moments : Subsystem
  Wind to body axis rotation : Subsystem
  Forces_total_BUS : Outport
  Moments_total_BUS : Outport  Port=2
  wires:
  Aero_Coefficients/2(Moment_Coeff_BUS) -> Total Aero Moments/3(Moment_Coeff_BUS)
  Aircraft_Constant_BUS/1 -> Total Aero Moments/2(Aircraft_Constants_BUS), Total Aero Forces/2(Aircraft_Constants_BUS), Aero_Coefficients/1(Aircraft_Constant_BUS)
  States with Wind/1(New_States_BUS) -> Aero_Coefficients/5(States_BUS), Wind to body axis rotation/3(States_BUS)
  Controls_BUS/1 -> Aero_Coefficients/3(Controls_BUS)
  Aero_Coefficients/1(Force_Coeff_BUS) -> Total Aero Forces/3(Force_Coeff_BUS)
  Atmosphere_BUS/1 -> Aero_Coefficients/2(Atmosphere_BUS), Total Aero Moments/1(Atmosphere_BUS), Total Aero Forces/1(Atmosphere_BUS)
  Total Aero Moments/1(Moments_total_BUS) -> Wind to body axis rotation/2(Moments_wind)
  Total Aero Forces/1(Forces_total_BUS) -> Wind to body axis rotation/1(Forces_wind)
  Engine_BUS/1 -> Aero_Coefficients/4(Engine_BUS)
  Wind to body axis rotation/1(Forces_body) -> Bus Selector/1, Scope/1, Forces_total_BUS/1
  Wind to body axis rotation/2(Moments_body) -> Bus Selector1/1, Scope1/1, Moments_total_BUS/1
  LE_Flaps_BUS/1 -> Terminator/1
  States_BUS/1 -> States with Wind/1(States_BUS)
  Vel_aero_BUS/1 -> States with Wind/2(Vel_aero_BUS)
  Bus Selector/1 -> Mux/1  "<X_total>"
  Bus Selector/2 -> Mux/2  "<Z_total>"
  Mux/1 -> To Workspace/1
  Bus Selector1/1 -> To Workspace1/1  "<M_total>"

== system Flight_Simulation/Non-linear_Plant/Engine_Model ==
  Command_BUS : Inport
  Flag_Settings_BUS : Inport  Port=2
  Init_BUS : Inport  Port=3
  Aircraft_Constants_BUS : Inport  Port=4
  Atmosphere_BUS : Inport  Port=5
  Bus Creator : BusCreator  Inputs=3
  Bus Selector : BusSelector  OutputSignals=Thrust_cmd_N
  Bus Selector1 : BusSelector  OutputSignals=U_init_BUS.Thrust_init_N
  Bus Selector2 : BusSelector  OutputSignals=Linearization_Flag
  Bus Selector3 : BusSelector  OutputSignals=q_bar_Pa
  Bus Selector4 : BusSelector  OutputSignals=Engine_Const_BUS
  Bus Selector7 : BusSelector  OutputSignals=z_eng
  Moment due to dZ_Engine : Product
  Propeller CT Calculation : Subsystem
  Switch : Switch  Criteria=u2 > Threshold
  Thrust Model : Subsystem
  Engine_BUS : Outport
  wires:
  Command_BUS/1 -> Bus Selector/1
  Bus Creator/1 -> Engine_BUS/1  "Engine_BUS"
  Aircraft_Constants_BUS/1 -> Bus Selector4/1
  Switch/1 -> Bus Creator/1, Moment due to dZ_Engine/1  "Thrust_act_N"
  Init_BUS/1 -> Bus Selector1/1
  Bus Selector1/1 -> Thrust Model/2(Thrust_init_N)  "<Thrust_init_N>"
  Thrust Model/1(Thrust_act_N) -> Switch/3  "Thrust_act_N"
  Flag_Settings_BUS/1 -> Bus Selector2/1
  Bus Selector2/1 -> Switch/2  "<Linearization_Flag>"
  Atmosphere_BUS/1 -> Bus Selector3/1
  Bus Selector/1 -> Propeller CT Calculation/1(Thrust_cmd_N), Switch/1, Thrust Model/1(Thrust_cmd_N)  "<Thrust_cmd_N>"
  Bus Selector3/1 -> Propeller CT Calculation/2(q_bar_Pa)  "<q_bar_Pa>"
  Propeller CT Calculation/1(CT) -> Bus Creator/2  "CT"
  Bus Selector4/1 -> Thrust Model/3(Aircraft_Constants_BUS), Propeller CT Calculation/3(Propeler_S_m^2), Bus Selector7/1  "<Engine_Const_BUS>"
  Bus Selector7/1 -> Moment due to dZ_Engine/2  "<z_eng>"
  Moment due to dZ_Engine/1 -> Bus Creator/3  "M_engine_Nm"

== system Flight_Simulation/State_Integration_pure_simulink/Calc_U_V_W ==
  Vel_aero_alpha_beta : Inport
  Bus Creator : BusCreator  Inputs=3
  Bus Selector1 : BusSelector  OutputSignals=v_m/s,alpha_rad,beta_rad
  Product : Product  Inputs=3
  Product1 : Product
  Product2 : Product  Inputs=3
  Trigonometric Function : Trigonometry
  Trigonometric Function1 : Trigonometry
  Trigonometric Function2 : Trigonometry  Operator=cos
  Trigonometric Function3 : Trigonometry  Operator=cos
  Vel_U_V_W : Outport
  wires:
  Trigonometric Function1/1 -> Product1/2  "sb"
  Trigonometric Function3/1 -> Product2/3, Product/3  "cb"
  Product/1 -> Bus Creator/1  "Vel_U_m/s"
  Bus Selector1/1 -> Product2/1, Product1/1, Product/1  "<v_m/s>"
  Trigonometric Function2/1 -> Product/2  "ca"
  Product1/1 -> Bus Creator/2  "Vel_V_m/s"
  Bus Selector1/3 -> Trigonometric Function1/1, Trigonometric Function3/1  "<beta_rad>"
  Trigonometric Function/1 -> Product2/2  "sa"
  Bus Selector1/2 -> Trigonometric Function/1, Trigonometric Function2/1  "<alpha_rad>"
  Product2/1 -> Bus Creator/3  "Vel_W_m/s"
  Vel_aero_alpha_beta/1 -> Bus Selector1/1
  Bus Creator/1 -> Vel_U_V_W/1  "Vel_U_V_W"

== system Flight_Simulation/State_Integration_pure_simulink/Vel_aero_dot_Calculation ==
  Vel_U_V_W_BUS : Inport
  States_BUS : Inport  Port=2
  Vel_U_V_W_dot_BUS : Inport  Port=3
  Bus Creator : BusCreator  Inputs=3
  Vel_aero_dot_total : Subsystem
  alpha_aero_dot : Subsystem
  beta_aero_dot : Subsystem
  Vel_aero_dot_V_alpha_beta_BUS : Outport
  wires:
  States_BUS/1 -> beta_aero_dot/1(States_BUS), alpha_aero_dot/1(States_BUS), Vel_aero_dot_total/1(States_BUS)
  Vel_U_V_W_BUS/1 -> alpha_aero_dot/2(Vel_U_V_W_BUS), beta_aero_dot/2(Vel_U_V_W_BUS), Vel_aero_dot_total/2(Vel_U_V_W_BUS)
  Vel_U_V_W_dot_BUS/1 -> beta_aero_dot/3(Vel_U_V_W_dot_BUS), alpha_aero_dot/3(Vel_U_V_W_dot_BUS), Vel_aero_dot_total/3(Vel_U_V_W_dot_BUS)
  Vel_aero_dot_total/1(V_aero_tot_dot) -> beta_aero_dot/4(V_aero_total_dot), Bus Creator/1
  Bus Creator/1 -> Vel_aero_dot_V_alpha_beta_BUS/1  "Vel_dot_aero_V_alpha_beta"
  alpha_aero_dot/1(alpha_aero_dot) -> Bus Creator/2
  beta_aero_dot/1(beta_aero_dot) -> Bus Creator/3

== system Flight_Simulation/Trim_Results/U_init_BusCreation ==
  Bus Creator : BusCreator  Inputs=4
  Constant : Constant  Value=Trim.Controls_result.Thrust(1)
  Constant1 : Constant  Value=Trim.Controls_result.Elevator(1)
  Constant2 : Constant  Value=Trim.Controls_result.Aileron(1)
  Constant3 : Constant  Value=Trim.Controls_result.Rudder(1)
  U_init_BUS : Outport
  wires:
  Bus Creator/1 -> U_init_BUS/1  "U_init_BUS"
  Constant1/1 -> Bus Creator/2  "Elevator_init_deg"
  Constant2/1 -> Bus Creator/3  "Aileron_init_deg"
  Constant3/1 -> Bus Creator/4  "Rudder_init_deg"
  Constant/1 -> Bus Creator/1  "Thrust_init_N"

== system Flight_Simulation/Trim_Results/X_init_BusCreation ==
  Bus Creator : BusCreator  Inputs=5
  Bus Creator{1..5} (5 alike) : BusCreator  Inputs=3
  Constant : Constant  Value=Trim.States_result.north_pos(1)
  Constant1 : Constant  Value=Trim.States_result.east_pos(1)
  Constant10 : Constant  Value=Trim.States_result.W(1)  VectorParams1D=off
  Constant11 : Constant  Value=Trim.States_result.p(1)  VectorParams1D=off
  Constant12 : Constant  Value=Trim.States_result.q(1)  VectorParams1D=off
  Constant13 : Constant  Value=Trim.States_result.r(1)  VectorParams1D=off
  Constant2 : Constant  Value=Trim.States_result.Altitude(1)
  Constant3 : Constant  Value=Trim.States_result.lambda(1)
  Constant4 : Constant  Value=Trim.States_result.mue(1)
  Constant5 : Constant  Value=Trim.States_result.phi(1)
  Constant6 : Constant  Value=Trim.States_result.theta(1)
  Constant7 : Constant  Value=Trim.States_result.psi(1)
  Constant8 : Constant  Value=Trim.States_result.U(1)
  Constant9 : Constant  Value=Trim.States_result.V(1)  VectorParams1D=off
  Gain : Gain  Gain=pi/180
  Gain1 : Gain  Gain=pi/180
  Gain2 : Gain
  X_init_BUS : Outport
  wires:
  Constant10/1 -> Bus Creator3/3  "W_init_m/s"
  Constant12/1 -> Bus Creator4/2  "q_init_rad/s"
  Constant/1 -> Bus Creator1/1  "north_pos_init_m"
  Constant1/1 -> Bus Creator1/2  "east_pos_init_m"
  Constant6/1 -> Bus Creator2/2  "theta_init_rad"
  Constant5/1 -> Bus Creator2/1  "phi_init_rad"
  Constant9/1 -> Bus Creator3/2  "V_init_m/s"
  Constant8/1 -> Bus Creator3/1  "U_init_m/s"
  Constant7/1 -> Bus Creator2/3  "psi_init_rad"
  Constant2/1 -> Gain2/1, Bus Creator1/3  "altitude_init_m"
  Constant11/1 -> Bus Creator4/1  "p_init_rad/s"
  Constant13/1 -> Bus Creator4/3  "r_init_rad/s"
  Bus Creator/1 -> X_init_BUS/1  "X_init_BUS"
  Bus Creator1/1 -> Bus Creator/1  "Position_north_east_alt_init"
  Bus Creator2/1 -> Bus Creator/2  "Angles_phi_theta_psi_init"
  Bus Creator3/1 -> Bus Creator/3  "U_V_W_body_init"
  Bus Creator4/1 -> Bus Creator/4  "Rates_p_q_r_init"
  Constant4/1 -> Gain1/1
  Gain/1 -> Bus Creator5/1  "lambda_WGS84_rad"
  Gain1/1 -> Bus Creator5/2  "mue_WGS84_rad"
  Gain2/1 -> Bus Creator5/3  "h_WGS84_m"
  Bus Creator5/1 -> Bus Creator/5  "Position_WGS84_init"
  Constant3/1 -> Gain/1

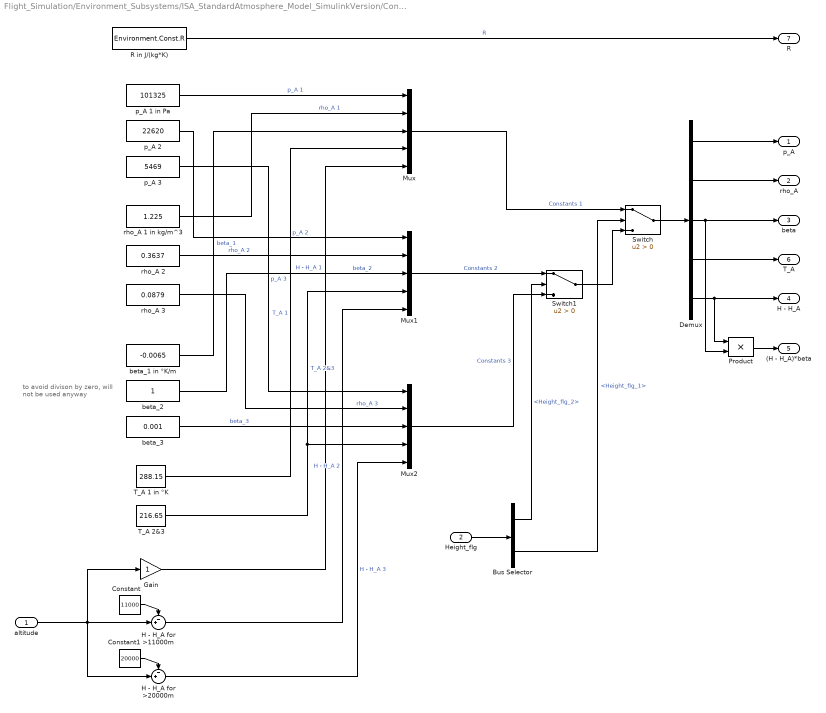
== system Flight_Simulation/Environment_Subsystems/ISA_StandardAtmosphere_Model_SimulinkVersion/Constants depending on Height ==
  note: to avoid divison by zero,
      | will not be used anyway
  altitude : Inport
  Height_flg : Inport  Port=2
  Bus Selector : BusSelector  OutputSignals=Height_flg_2,Height_flg_1
  Constant : Constant  Value=11000
  Constant1 : Constant  Value=20000
  Demux : Demux  Outputs=5
  Gain : Gain
  H - H_A for >11000m : Sum  Inputs=-+|
  H - H_A for >20000m : Sum  Inputs=-+|
  Mux : Mux  Inputs=5
  Mux1 : Mux  Inputs=5
  Mux2 : Mux  Inputs=5
  Product : Product
  R in J/(kg*K) : Constant  Value=Environment.Const.R
  Switch : Switch  Criteria=u2 > Threshold
  Switch1 : Switch  Criteria=u2 > Threshold
  T_A 1 in °K : Constant  Value=288.15
  T_A 2&3 : Constant  Value=216.65
  beta_1 in °K/m : Constant  Value=-0.0065
  beta_2 : Constant
  beta_3 : Constant  Value=0.001
  p_A 1 in Pa : Constant  Value=101325
  p_A 2 : Constant  Value=22620
  p_A 3 : Constant  Value=5469
  rho_A 1 in kg/m^3 : Constant  Value=1.225
  rho_A 2 : Constant  Value=0.3637
  rho_A 3 : Constant  Value=0.0879
  p_A : Outport
  rho_A : Outport  Port=2
  beta : Outport  Port=3
  H - H_A : Outport  Port=4
  (H - H_A)*beta : Outport  Port=5
  T_A : Outport  Port=6
  R : Outport  Port=7
  wires:
  p_A 1 in Pa/1 -> Mux/1  "p_A 1"
  beta_1 in °K/m/1 -> Mux/3  "beta_1"
  T_A 1 in °K/1 -> Mux/4  "T_A 1"
  beta_3/1 -> Mux2/3  "beta_3"
  p_A 2/1 -> Mux1/1  "p_A 2"
  rho_A 1 in kg/m^3/1 -> Mux/2  "rho_A 1"
  p_A 3/1 -> Mux2/1  "p_A 3"
  rho_A 2/1 -> Mux1/2  "rho_A 2"
  rho_A 3/1 -> Mux2/2  "rho_A 3"
  T_A 2&3/1 -> Mux1/4, Mux2/4  "T_A 2&3"
  R in J/(kg*K)/1 -> R/1  "R"
  Height_flg/1 -> Bus Selector/1
  Bus Selector/2 -> Switch/2  "<Height_flg_1>"
  Switch1/1 -> Switch/3
  Bus Selector/1 -> Switch1/2  "<Height_flg_2>"
  Mux/1 -> Switch/1  "Constants 1"
  beta_2/1 -> Mux1/3  "beta_2"
  Mux1/1 -> Switch1/1  "Constants 2"
  Mux2/1 -> Switch1/3  "Constants 3"
  Switch/1 -> Demux/1
  Demux/1 -> p_A/1
  Demux/4 -> T_A/1
  Demux/3 -> beta/1, Product/2
  Demux/2 -> rho_A/1
  Constant1/1 -> H - H_A for >20000m/1
  Constant/1 -> H - H_A for >11000m/1
  Gain/1 -> Mux/5  "H - H_A 1"
  H - H_A for >11000m/1 -> Mux1/5  "H - H_A 2"
  H - H_A for >20000m/1 -> Mux2/5  "H - H_A 3"
  altitude/1 -> Gain/1, H - H_A for >20000m/2, H - H_A for >11000m/2
  Demux/5 -> H - H_A/1, Product/1
  Product/1 -> (H - H_A)*beta/1

== system Flight_Simulation/Environment_Subsystems/ISA_StandardAtmosphere_Model_SimulinkVersion/Height flags ==
  altitude : Inport
  Bus Creator1 : BusCreator  Inputs=2
  Compare To Constant : simulink/Logic and Bit Operations/Compare To Constant  relop=<  const=11000  OutDataTypeStr=boolean
  Compare To Constant1 : simulink/Logic and Bit Operations/Compare To Constant  relop=>  const=20000  OutDataTypeStr=boolean
  NOR : Logic  Operator=NOR  IconShape=distinctive  AllPortsSameDT=off  OutDataTypeStr=boolean
  Height_flg : Outport
  wires:
  Compare To Constant1/1 -> NOR/2  "Height_flg_3"
  altitude/1 -> Compare To Constant1/1, Compare To Constant/1
  NOR/1 -> Bus Creator1/2  "Height_flg_2"
  Compare To Constant/1 -> NOR/1, Bus Creator1/1  "Height_flg_1"
  Bus Creator1/1 -> Height_flg/1  "Height_flg"

== system Flight_Simulation/Environment_Subsystems/ISA_StandardAtmosphere_Model_SimulinkVersion/Mach ==
  note: a
  T : Inport
  R : Inport  Port=2
  v : Inport  Port=3
  Divide : Product  Inputs=/*
  Product : Product
  Sqrt : Sqrt  SaturateOnIntegerOverflow=on
  kappa : Gain  Gain=1.4
  Mach : Outport
  wires:
  Product/1 -> Sqrt/1
  Divide/1 -> Mach/1  "Mach"
  v/1 -> Divide/2
  kappa/1 -> Product/1
  Sqrt/1 -> Divide/1
  T/1 -> kappa/1
  R/1 -> Product/2

== system Flight_Simulation/Environment_Subsystems/ISA_StandardAtmosphere_Model_SimulinkVersion/T ==
  (H - H_A)*beta : Inport
  T_A : Inport  Port=2
  Height_flg : Inport  Port=3
  Add : Sum
  Bus Selector1 : BusSelector  OutputSignals=Height_flg_2
  Switch : Switch  Criteria=u2 > Threshold
  T : Outport
  wires:
  Bus Selector1/1 -> Switch/2  "<Height_flg_2>"
  Switch/1 -> T/1  "T"
  Add/1 -> Switch/3
  T_A/1 -> Add/1, Switch/1
  (H - H_A)*beta/1 -> Add/2
  Height_flg/1 -> Bus Selector1/1

== system Flight_Simulation/Environment_Subsystems/ISA_StandardAtmosphere_Model_SimulinkVersion/p_static ==
  p_A : Inport
  beta : Inport  Port=2
  H - H_A : Inport  Port=3
  (H - H_A)*beta : Inport  Port=4
  T_A : Inport  Port=5
  Height_flg : Inport  Port=6
  -g/R : Inport  Port=7
  *(-g/R) : Product
  *p_A : Product
  *p_A1 : Product
  Add : Sum
  Bus Selector3 : BusSelector  OutputSignals=Height_flg_2
  Constant : Constant
  Divide1 : Product  Inputs=*/
  Divide2 : Product  Inputs=*/
  Divide3 : Product  Inputs=*/
  Exp : Math  SaturateOnIntegerOverflow=on
  Math Function : Math  Operator=pow  SaturateOnIntegerOverflow=on
  Switch : Switch  Criteria=u2 > Threshold
  p : Outport
  wires:
  Math Function/1 -> *p_A1/2
  T_A/1 -> Divide2/2, Divide1/2
  beta/1 -> Divide3/2
  Add/1 -> Math Function/1
  (H - H_A)*beta/1 -> Divide2/1
  *(-g/R)/1 -> Exp/1
  Divide2/1 -> Add/1
  Exp/1 -> *p_A/1
  Divide1/1 -> *(-g/R)/1
  Constant/1 -> Add/2
  p_A/1 -> *p_A1/1, *p_A/2
  Divide3/1 -> Math Function/2
  H - H_A/1 -> Divide1/1
  Height_flg/1 -> Bus Selector3/1
  *p_A/1 -> Switch/1
  Switch/1 -> p/1
  Bus Selector3/1 -> Switch/2  "<Height_flg_2>"
  -g/R/1 -> Divide3/1, *(-g/R)/2
  *p_A1/1 -> Switch/3

== system Flight_Simulation/Environment_Subsystems/ISA_StandardAtmosphere_Model_SimulinkVersion/q_bar ==
  p_static : Inport
  rho : Inport  Port=2
  v : Inport  Port=3
  Mach : Inport  Port=4
  (k-1) : Sum  Inputs=+-
  (k-1)/2 : Gain  Gain=1/2
  Add : Sum
  Compressibility_Setting : Constant  Value=Settings.Compressibility
  Constant : Constant  Value=Environment.Const.k
  Constant2 : Constant
  Constant3 : Constant
  Constant4 : Constant  Value=2
  Constant5 : Constant
  Gain3 : Gain  Gain=0.5
  Mach^2 : Math  Operator=square  SaturateOnIntegerOverflow=on
  Math Function1 : Math  Operator=pow  SignedPower=on  SaturateOnIntegerOverflow=on
  NOT : Logic  Operator=NOT  IconShape=distinctive  AllPortsSameDT=off  OutDataTypeStr=boolean
  Power : Math  Operator=pow  SaturateOnIntegerOverflow=on
  Product : Product
  Product1 : Product
  Product2 : Product
  Subtract2 : Sum  Inputs=+-
  Switch : Switch  Criteria=u2 > Threshold
  k/(k-1) : Product  Inputs=*/
  q_bar : Outport
  wires:
  v/1 -> Math Function1/1
  Gain3/1 -> Product2/1
  Math Function1/1 -> Product2/2
  Constant4/1 -> Math Function1/2
  rho/1 -> Gain3/1
  Product2/1 -> Switch/1  "q_bar_Pa"
  Compressibility_Setting/1 -> NOT/1
  p_static/1 -> Product/1
  Mach/1 -> Mach^2/1
  Mach^2/1 -> Product1/2
  (k-1)/1 -> (k-1)/2/1, k/(k-1)/2
  (k-1)/2/1 -> Product1/1
  Product1/1 -> Add/2
  Add/1 -> Power/1
  Constant2/1 -> Add/1
  Constant3/1 -> (k-1)/2
  Constant/1 -> (k-1)/1, k/(k-1)/1
  k/(k-1)/1 -> Power/2
  Power/1 -> Subtract2/1
  Constant5/1 -> Subtract2/2
  Subtract2/1 -> Product/2
  Product/1 -> Switch/3  "q_bar_Pa"
  Switch/1 -> q_bar/1  "q_bar_Pa"
  NOT/1 -> Switch/2

== system Flight_Simulation/Environment_Subsystems/ISA_StandardAtmosphere_Model_SimulinkVersion/rho ==
  rho_A : Inport
  beta : Inport  Port=2
  H - H_A : Inport  Port=3
  (H - H_A)*beta : Inport  Port=4
  T_A : Inport  Port=5
  Height_flg : Inport  Port=6
  -g/R : Inport  Port=7
  *(-g/R) : Product
  *rho_A : Product
  *rho_A1 : Product
  Add : Sum
  Add1 : Sum  Inputs=+-
  Bus Selector3 : BusSelector  OutputSignals=Height_flg_2
  Constant : Constant
  Constant1 : Constant
  Divide1 : Product  Inputs=*/
  Divide2 : Product  Inputs=*/
  Divide3 : Product  Inputs=*/
  Exp : Math  SaturateOnIntegerOverflow=on
  Math Function : Math  Operator=pow  SaturateOnIntegerOverflow=on
  Switch : Switch  Criteria=u2 > Threshold
  rho : Outport
  wires:
  T_A/1 -> Divide2/2, Divide1/2
  *(-g/R)/1 -> Exp/1
  Exp/1 -> *rho_A/1
  Divide1/1 -> *(-g/R)/1
  Bus Selector3/1 -> Switch/2  "<Height_flg_2>"
  H - H_A/1 -> Divide1/1
  *rho_A/1 -> Switch/1
  Height_flg/1 -> Bus Selector3/1
  rho_A/1 -> *rho_A1/1, *rho_A/2
  Switch/1 -> rho/1
  -g/R/1 -> Divide3/1, *(-g/R)/2
  (H - H_A)*beta/1 -> Divide2/1
  Divide2/1 -> Add/1
  Constant/1 -> Add/2
  beta/1 -> Divide3/2
  Constant1/1 -> Add1/2
  Divide3/1 -> Add1/1
  Add/1 -> Math Function/1
  Add1/1 -> Math Function/2
  Math Function/1 -> *rho_A1/2
  *rho_A1/1 -> Switch/3
